simulink model "Temperaturregelung"  (R2021b)
settings: Solver=ode3  StartTime=0.0  StopTime=10.0  FixedStep=0.01  RelTol=1e-3
undefined symbols (not defined in the file or in its folder): sigbuilder_block
settings Model: Creator=mwjae  LastModifiedBy=mwjae

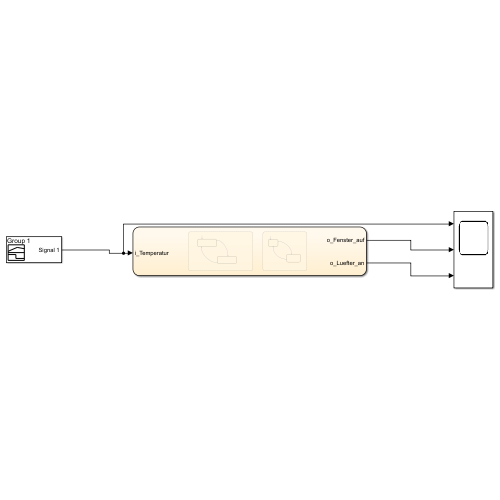
[thumbnail: Simulink's stored preview of the top-level diagram]
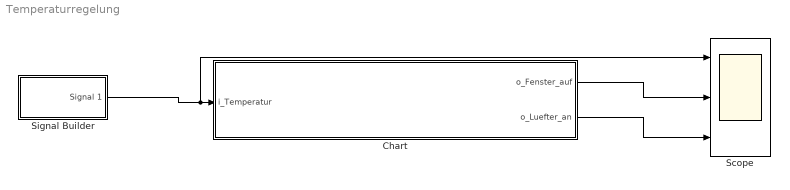
== system Temperaturregelung ==
  Chart : Stateflow chart  TreatAsAtomicUnit=on
  Scope : Scope  NumInputPorts=3
  Signal Builder : Subsystem  Tag=STV Subsys  LoadFcn=sigbuilder_block('load');  StartFcn=sigbuilder_block('start');  StopFcn=sigbuilder_block('stop');  ClipboardFcn=sigbuilder_block('clipboard');  mask(Sigbuilder block){tuvar=[0:10]}
      mask help: Simulink:masks:SigbuilderBlock_MD
      mask init:
      | if ~strcmp(get_param(bdroot(gcbh),'SimulationStatus'),'stopped') tuvar = sigbuilder_block('maskInit'); end
      settings: CopyFcn=sigbuilder_block('copy');  DeleteFcn=sigbuilder_block('delete');  ModelCloseFcn=sigbuilder_block('modelClose');  PreSaveFcn=sigbuilder_block('preSave');  PauseFcn=sigbuilder_block('pause');  ContinueFcn=sigbuilder_block('continue');  NameChangeFcn=sigbuilder_block('namechange');  OpenFcn=sigbuilder_block('open',[153 199.5 550.5 399.75 ]);  CloseFcn=sigbuilder_block('close');
      mask Display: plot(0, 0, 100, 100,[2, 2, 32, 32, 2], [68, 8, 8, 68, 68],[32, 2], [38, 38], [32, 19, 2],[53, 60, 44], [32, 17, 17, 2],[16, 16, 31, 31]);txt = getActiveGroup(gcbh);text(2, 100, txt,'verticalAlignment', 'top');
  wires:
  Signal Builder/1(Signal 1) -> Scope/1, Chart/1(i_Temperatur)
  Chart/1(o_Fenster_auf) -> Scope/2
  Chart/2(o_Luefter_an) -> Scope/3

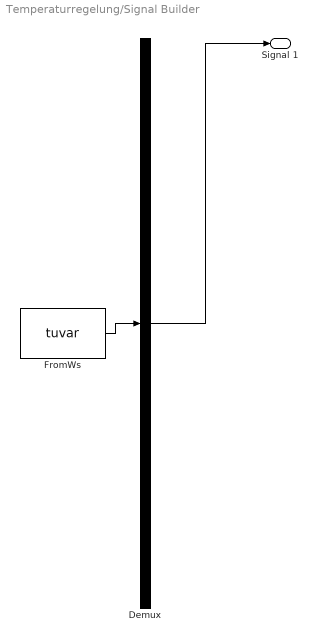
== system Temperaturregelung/Signal Builder ==
  Demux : Demux  Tag=STV Demux  Outputs=1
      settings: DisplayOption=none
  FromWs : FromWorkspace  Tag=STV FromWs  VariableName=tuvar
      SigBuilderData=|
      | common.afterFinalStr = 'Extrapolate'
      | common.sampleTime = 0
      | dataSet.timeRange = [0 10]
      | dataSet.name = 'Group 1'
      | sbobj.Groups.Name = 'Group 1'
      | sbobj.Groups.Signals.Name = 'Signal 1'
      | sbobj.Groups.Signals.XData = [0 1 1 2 2 4 4 6 6 10]
      | sbobj.Groups.Signals.YData = [15 15 17.6 21.8 25.4 40.4 7.8 10.8 36.4 17.4]
  Signal 1 : Outport  Tag=STV Outport
  wires:
  Demux/1 -> Signal 1/1
  FromWs/1 -> Demux/1

== stateflow chart Temperaturregelung/Chart ==
  state Fenster [parallel]
    settings: executionOrder=1
    state Fester_close
    state Fester_open
    (default) -> Fester_close
    Fester_close -> Fester_open : [i_Temperatur>25]{o_Fenster_auf=1}
    Fester_open -> Fester_close : [i_Temperatur <20]{o_Fenster_auf =0}
  state Luefter [parallel]
    settings: executionOrder=2
    state Luefter_close
    state Luefter_open
    (default) -> Luefter_close
    Luefter_close -> Luefter_open : [i_Temperatur > 30]{o_Luefter_an =1}
    Luefter_open -> Luefter_close : [i_Temperatur < 25]{o_Luefter_an = 0}
  data: i_Temperatur input; o_Fenster_auf output; o_Luefter_an output
